simulink model "Line2GotoFromDemo"  (Simulink 7.8)
settings: Solver=ode45  StartTime=0.0  StopTime=10.0  RelTol=1e-3
settings Model: Creator=T6684MB  LastModifiedBy=monika

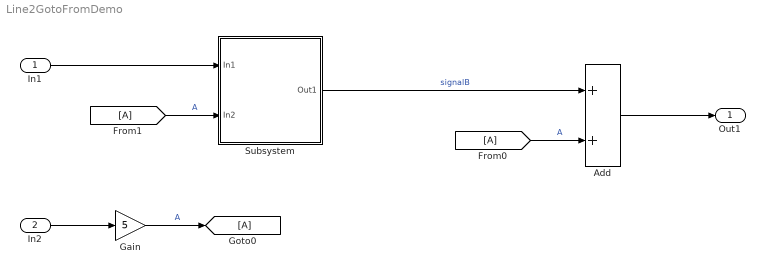
== system Line2GotoFromDemo ==
  In1 : Inport
  In2 : Inport  Port=2
  Add : Sum
  Gain : Gain  Gain=5
  Subsystem : Subsystem
  Out1 : Outport
  wires:
  Add/1 -> Out1/1
  In2/1 -> Gain/1
  In1/1 -> Subsystem/1(In1)
  Subsystem/1(Out1) -> Add/1  "signalB"
  Gain/1 -> [A]  "A"
  [A] -> Add/2  "A"
  [A] -> Subsystem/2(In2)  "A"

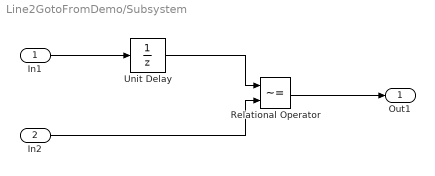
== system Line2GotoFromDemo/Subsystem ==
  In1 : Inport
  In2 : Inport  Port=2
  Relational Operator : RelationalOperator  Operator=~=  OutDataTypeStr=boolean
  Unit Delay : UnitDelay  SampleTime=-1
  Out1 : Outport
  wires:
  In1/1 -> Unit Delay/1
  Unit Delay/1 -> Relational Operator/1
  In2/1 -> Relational Operator/2
  Relational Operator/1 -> Out1/1
